simulink model "skok"  (R2018b)
settings: Solver=VariableStepAuto  StartTime=0.0  StopTime=30  RelTol=1e-3
values from neighbouring files (symbols this model uses):
  a = aS(i)    [odpskokowe.m]
  b = bS(i)    [odpskokowe.m]
settings Model: Creator=Witaj Przemku  LastModifiedBy=lev
settings SFSimCC: SimUseLocalCustomCode=off
settings RTWCC: RTWUseLocalCustomCode=off
settings CodeAppCC: StateflowObjectComments=on

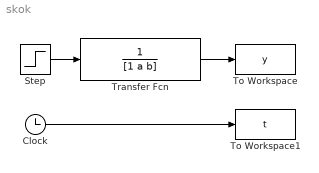
== system skok ==
  Clock : Clock
  Step : Step  Time=0  SampleTime=0
  To Workspace : ToWorkspace  VariableName=y  SampleTime=0.01
      settings: Save2DSignal=2-D array (concatenate along first dimension)
  To Workspace1 : ToWorkspace  VariableName=t  SampleTime=0.01
      settings: Save2DSignal=2-D array (concatenate along first dimension)
  Transfer Fcn : TransferFcn  Denominator=[1 a b]
  wires:
  Transfer Fcn/1 -> To Workspace/1
  Clock/1 -> To Workspace1/1
  Step/1 -> Transfer Fcn/1
